simulink model "quadrotor_1d_nonlin"  (R2020a)
settings: Solver=VariableStepAuto  StartTime=0.0  StopTime=20  RelTol=1e-3
undefined symbols (not defined in the file): m
libraries: simulink x1
settings Model: Creator=janusboandersen  LastModifiedBy=janusboandersen

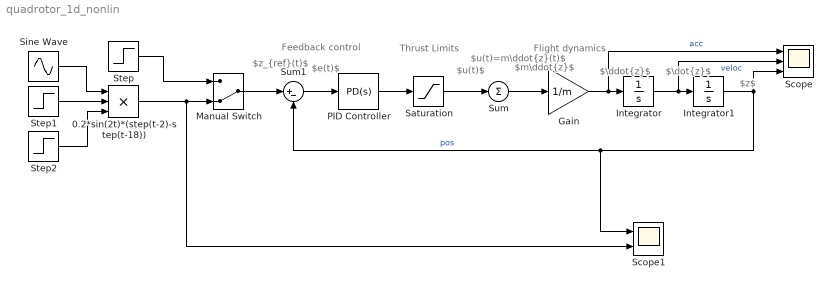
== system quadrotor_1d_nonlin ==
  note: Thrust
      | Limits
  note: Flight
      | dynamics
  note: $m\ddot{z}$
  note: $u(t)=m\ddot{z}(t)$
  note: $\ddot{z}$
  note: $\dot{z}$
  note: $z$
  note: $u(t)$
  note: $e(t)$
  note: $z_{ref}(t)$
  note: Feedback
      | control
  0.2*sin(2t)*(step(t-2)-step(t-18)) : Product  Inputs=3
  Gain : Gain  Gain=1/m
  Integrator : Integrator
  Integrator1 : Integrator
  Manual Switch : ManualSwitch  CurrentSetting=0
  PID Controller : simulink/Continuous/PID Controller  Controller=PD  Form=Parallel  TimeDomain=Continuous-time  UseExternalTs=off  SampleTime=-1  IntegratorMethod=Forward Euler  FilterMethod=Forward Euler  ControllerParametersSource=internal  P=0.811387890066875  I=0  D=0.487634074944938  UseFilter=on  N=109.108960288243  TunerSelectOption=Transfer Function Based (PID Tuner App)  InitialConditionSource=internal  InitialConditionForIntegrator=0  InitialConditionForFilter=0  DifferentiatorICPrevScaledInput=0  ExternalReset=none  TrackingMode=off  Kt=1  LimitOutput=off  UpperSaturationLimit=inf  LowerSaturationLimit=-inf  LinearizeAsGain=on  AntiWindupMode=none  Kb=1  POutMin=[]  POutMax=[]  IOutMin=[]  IOutMax=[]  DOutMin=[]  DOutMax=[]  NOutMin=[]  NOutMax=[]  SumOutMin=[]  SumOutMax=[]  SaturationOutMin=[]  SaturationOutMax=[]  PParamMin=[]  PParamMax=[]  IParamMin=[]  IParamMax=[]  DParamMin=[]  DParamMax=[]  NParamMin=[]  NParamMax=[]  KbParamMin=[]  KbParamMax=[]  KtParamMin=[]  KtParamMax=[]  KbOutMin=[]  KbOutMax=[]  KtOutMin=[]  KtOutMax=[]  IntegratorOutMin=[]  IntegratorOutMax=[]  FilterOutMin=[]  FilterOutMax=[]  SumI1OutMin=[]  SumI1OutMax=[]  SumI2OutMin=[]  SumI2OutMax=[]  SumI3OutMin=[]  SumI3OutMax=[]  SumI4OutMin=[]  SumI4OutMax=[]  SumDOutMin=[]  SumDOutMax=[]  DifferentiatorOutMin=[]  DifferentiatorOutMax=[]  FilterDiffOutCoefMin=[]  FilterDiffOutCoefMax=[]  ReciprocalOutMin=[]  ReciprocalOutMax=[]  SumDenOutMin=[]  SumDenOutMax=[]  SumNumOutMin=[]  SumNumOutMax=[]  DivideOutMin=[]  DivideOutMax=[]  UdiffTsProdOutMin=[]  UdiffTsProdOutMax=[]  NTsProdOutMin=[]  NTsProdOutMax=[]  UintegralTsProdOutMin=[]  UintegralTsProdOutMax=[]  UngainTsProdOutMin=[]  UngainTsProdOutMax=[]  IntegratorContinuousStateAttributes=''  IntegratorStateMustResolveToSignalObject=off  IntegratorRTWStateStorageClass=Auto  FilterContinuousStateAttributes=''  FilterStateMustResolveToSignalObject=off  FilterRTWStateStorageClass=Auto  ParallelPVariant=InternalParameters  IdealPVariant=Disabled  IVariant=Disabled  DVariant=InternalParameters  IntegratorVariant=Disabled  SatVariant=Disabled  AWVariant=Disabled  PCopyVariant=Disabled  TRVariant=Disabled  FdbkBlocksVariant=Forward  IdealPFdbkVariant=Disabled  SatFdbkVariant=Disabled  DerivativeFilterVariant=ContFilter  NVariant=InternalParameters  NCopyVariant=Disabled  FilterICVariant=InternalICsFilter  IntegratorICVariant=Disabled  ExternalResetVariant=Disabled  TRSumVariant=Passthrough  SumFdbkVariant=Disabled  SumVariant=Sum_PD  TsampFilterVariant=InternalTs  TsampNgainVariant=Passthrough  TsampIntegralVariant=Disabled_SignalSpec
  Saturation : Saturate  UpperLimit=0.38  LowerLimit=-0.62
  Scope : Scope  NumInputPorts=3
  Scope1 : Scope  NumInputPorts=2
  Sine Wave : Sin  Amplitude=0.2  Bias=1  Frequency=2  SampleTime=0
  Step : Step  Time=0  SampleTime=0
  Step1 : Step  Time=2  SampleTime=0
  Step2 : Step  Time=18  Before=1  After=0  SampleTime=0
  Sum : Sum  Inputs=+
  Sum1 : Sum  Inputs=|+-
  wires:
  Sum/1 -> Gain/1
  Integrator/1 -> Scope/2, Integrator1/1  "veloc"
  Integrator1/1 -> Scope1/1, Sum1/2, Scope/3  "pos"
  Sum1/1 -> PID Controller/1
  Gain/1 -> Scope/1, Integrator/1  "acc"
  Saturation/1 -> Sum/1
  PID Controller/1 -> Saturation/1
  Sine Wave/1 -> 0.2*sin(2t)*(step(t-2)-step(t-18))/1
  Step1/1 -> 0.2*sin(2t)*(step(t-2)-step(t-18))/2
  0.2*sin(2t)*(step(t-2)-step(t-18))/1 -> Scope1/2, Manual Switch/2
  Step2/1 -> 0.2*sin(2t)*(step(t-2)-step(t-18))/3
  Step/1 -> Manual Switch/1
  Manual Switch/1 -> Sum1/1
